simulink model "Simulator_swintheloop"  (R2016a)
settings: Solver=ode45  StartTime=0.0  StopTime=sim_time  RelTol=1e-3
values from neighbouring files (symbols this model uses):
  A_Servo = [0 1 0; 0 0 1 ; -B4/B1 -B3/B1 -B2/B1]    [Parameters.m]
  B_Servo = [0 ; 0 ; B0/B1]    [Parameters.m]
  C_Servo = eye(3)    [Parameters.m]
  delay_Kaltitude = 1    [Parameters.m]
  dLMN = [dLdp  0    0 ... (first row only)    [Parameters.m]
  g = 9.81    [Parameters.m]
  I_Pi = diag([8.450e-5 8.450e-5 4.580e-5])    [Parameters.m]
  In = diag([Ixx Iyy Izz])    [Parameters.m]
  InInv = In\eye(3)    [Parameters.m]
  KaD = 5.4    [Parameters.m]
  KaI = 3.6    [Parameters.m]
  KaN = 38    [Parameters.m]
  KaP = 8.0    (= 8)    [Parameters.m]
  Kba = sqrt(KaD/KaI)    [Parameters.m]
  Kbp = sqrt(Kdp/Kip)    [Parameters.m]
  Kbq = sqrt(Kdq/Kiq)    [Parameters.m]
  Kbr = sqrt(Kdr/Kir)    [Parameters.m]
  Kd_E = Kd_N    (= 0.01)    [Parameters.m]
  Kd_N = 0.01    [Parameters.m]
  Kd_u = Kd_v    (= 0.29)    [Parameters.m]
  Kd_v = 0.290    (= 0.29)    [Parameters.m]
  Kdp = 0.006    [Parameters.m]
  Kdq = Kdp    (= 0.006)    [Parameters.m]
  Kdr = 0.0153    [Parameters.m]
  Kinv = wpinv(K,W)    [Parameters.m]
  Kip = 0.72    [Parameters.m]
  Kiq = Kip    (= 0.72)    [Parameters.m]
  Kir = 0.125    [Parameters.m]
  Kp_E = Kp_N    (= 0.15)    [Parameters.m]
  Kp_N = 0.15    [Parameters.m]
  Kp_u = Kp_v    (= 6.3)    [Parameters.m]
  Kp_v = 6.3    [Parameters.m]
  KPD = KRD    (= 0.0584)    [Parameters.m]
  KPP = KRP    (= 1.61)    [Parameters.m]
  Kpp = 0.3    [Parameters.m]
  Kpq = Kpp    (= 0.3)    [Parameters.m]
  Kpr = 0.135    [Parameters.m]
  Kq = Cq*ro*A*R^3    (= 2.88925724261e-07)    [Parameters.m]
  KRD = 0.0584    [Parameters.m]
  KRP = 1.61    [Parameters.m]
  Kt = Ct*ro*A*R^2    (= 2.46191978476e-05)    [Parameters.m]
  m = 1.900    (= 1.9)    [Parameters.m]
  Mb = diag([m m m])    [Parameters.m]
  MbInv = Mb\eye(3)    [Parameters.m]
  N = 1/Tf    (= 100)    [Parameters.m]
  N_tras = 100    [Parameters.m]
  pitchMax = pi/6    (= 0.523598775598)    [Parameters.m]
  rollMax = pi/6    (= 0.523598775598)    [Parameters.m]
  satp = 1.5    [Parameters.m]
  satq = 1.5    [Parameters.m]
  satr = 1    [Parameters.m]
  tau = 0.055257    [Parameters.m]
  tc = 1/fc    (= 0.01)    [Parameters.m]
  x1 = [m q]    [Parameters.m]
  yawRateMax = pi/2    (= 1.57079632679)    [Parameters.m]
undefined symbols (not defined in the file or in its folder): Kp, KPI, KRI
libraries: simulink x10, aerolibutil x10
(part 2 of 2)

== system Simulator_swintheloop/TiltCopter/Actuators/Traslational Force_2 ==
  alpha_i : Inport
  omega_i : Inport  Port=2
  Product : Product  Multiplication=Matrix(*)
  R_BP2 : MATLAB Function  TreatAsAtomicUnit=on
  Thrust computation : Subsystem
  F_i : Outport
  wires:
  Thrust computation/1(Vector_Thrust_i) -> Product/2
  Product/1 -> F_i/1
  omega_i/1 -> Thrust computation/1(omega_i)
  R_BP2/1(Rotation_matrix) -> Product/1
  alpha_i/1 -> R_BP2/1(alpha_2)

== system Simulator_swintheloop/TiltCopter/Actuators/Traslational Force_3 ==
  alpha_i : Inport
  omega_i : Inport  Port=2
  Product : Product  Multiplication=Matrix(*)
  R_BP3 : MATLAB Function  TreatAsAtomicUnit=on
  Thrust computation : Subsystem
  F_i : Outport
  wires:
  Thrust computation/1(Vector_Thrust_i) -> Product/2
  Product/1 -> F_i/1
  omega_i/1 -> Thrust computation/1(omega_i)
  R_BP3/1(Rotation_matrix) -> Product/1
  alpha_i/1 -> R_BP3/1(alpha_3)

== system Simulator_swintheloop/TiltCopter/Actuators/Traslational Force_4 ==
  alpha_i : Inport
  omega_i : Inport  Port=2
  Product : Product  Multiplication=Matrix(*)
  R_BP4 : MATLAB Function  TreatAsAtomicUnit=on
  Thrust computation : Subsystem
  F_i : Outport
  wires:
  Thrust computation/1(Vector_Thrust_i) -> Product/2
  Product/1 -> F_i/1
  omega_i/1 -> Thrust computation/1(omega_i)
  R_BP4/1(Rotation_matrix) -> Product/1
  alpha_i/1 -> R_BP4/1(alpha_4)

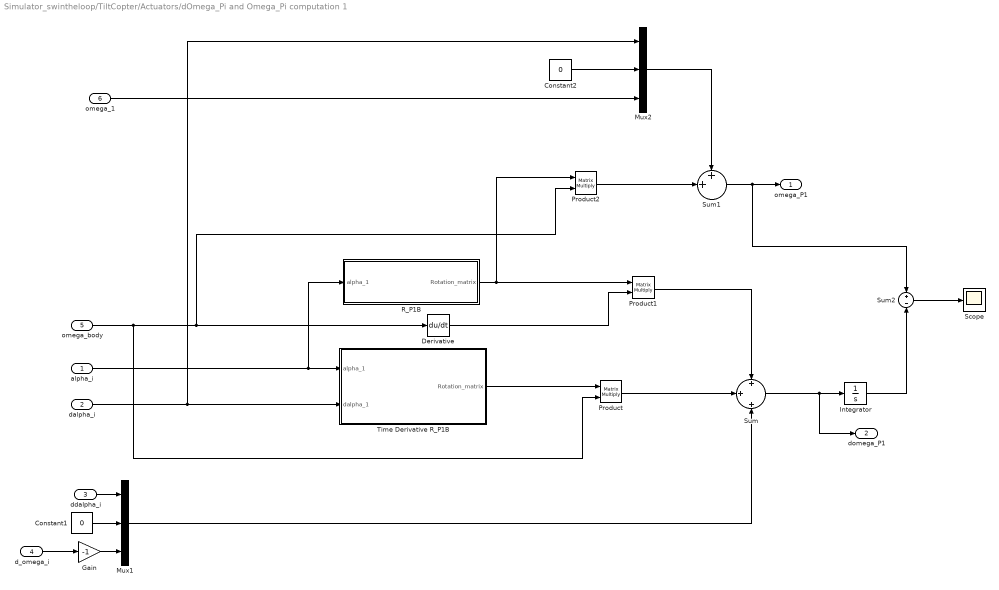
== system Simulator_swintheloop/TiltCopter/Actuators/dOmega_Pi and Omega_Pi computation 1 ==
  alpha_i : Inport
  dalpha_i : Inport  Port=2
  ddalpha_i : Inport  Port=3
  d_omega_i : Inport  Port=4
  omega_body : Inport  Port=5
  omega_1 : Inport  Port=6
  Constant1 : Constant  Value=0
  Constant2 : Constant  Value=0
  Derivative : Derivative
  Gain : Gain  Gain=-1
  Integrator : Integrator
  Mux1 : Mux  Inputs=3
  Mux2 : Mux  Inputs=3
  Product : Product  Multiplication=Matrix(*)
  Product1 : Product  Multiplication=Matrix(*)
  Product2 : Product  Multiplication=Matrix(*)
  R_P1B : MATLAB Function  TreatAsAtomicUnit=on
  Scope : Scope
  Sum : Sum  Inputs=+|+|+
  Sum1 : Sum  Inputs=++|
  Sum2 : Sum  Inputs=+-
  Time Derivative R_P1B : MATLAB Function  TreatAsAtomicUnit=on
  omega_P1 : Outport
  domega_P1 : Outport  Port=2
  wires:
  Derivative/1 -> Product1/2
  Product/1 -> Sum/2
  Time Derivative R_P1B/1(Rotation_matrix) -> Product/1
  Constant1/1 -> Mux1/2
  omega_body/1 -> Product/2, Product2/2, Derivative/1
  dalpha_i/1 -> Mux2/1, Time Derivative R_P1B/2(dalpha_1)
  alpha_i/1 -> R_P1B/1(alpha_1), Time Derivative R_P1B/1(alpha_1)
  R_P1B/1(Rotation_matrix) -> Product2/1, Product1/1
  Sum/1 -> domega_P1/1, Integrator/1
  Product1/1 -> Sum/1
  Mux1/1 -> Sum/3
  ddalpha_i/1 -> Mux1/1
  Product2/1 -> Sum1/2
  Constant2/1 -> Mux2/2
  Mux2/1 -> Sum1/1
  Sum1/1 -> Sum2/1, omega_P1/1
  omega_1/1 -> Mux2/3
  d_omega_i/1 -> Gain/1
  Integrator/1 -> Sum2/2
  Sum2/1 -> Scope/1
  Gain/1 -> Mux1/3

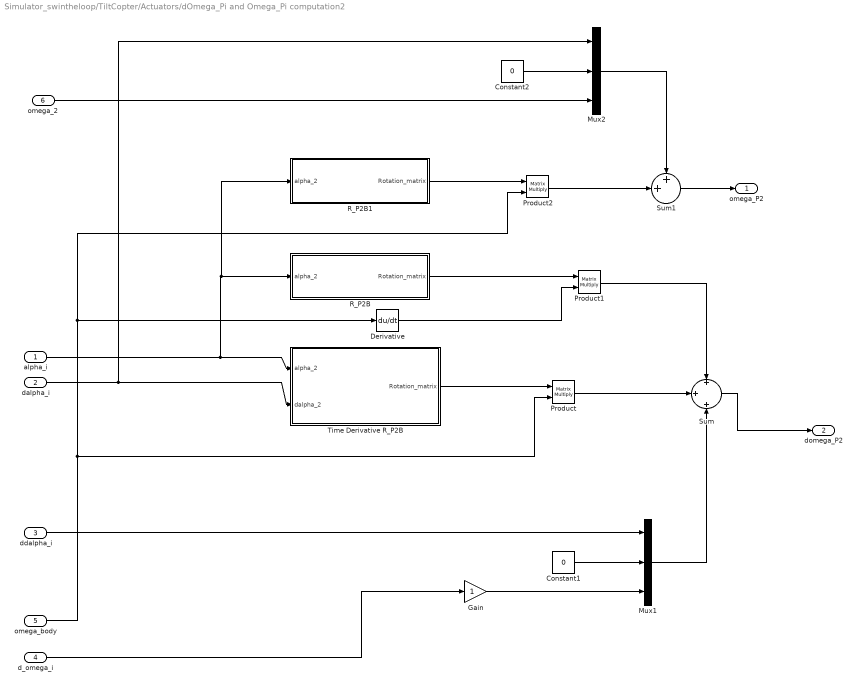
== system Simulator_swintheloop/TiltCopter/Actuators/dOmega_Pi and Omega_Pi computation2 ==
  alpha_i : Inport
  dalpha_i : Inport  Port=2
  ddalpha_i : Inport  Port=3
  d_omega_i : Inport  Port=4
  omega_body : Inport  Port=5
  omega_2 : Inport  Port=6
  Constant1 : Constant  Value=0
  Constant2 : Constant  Value=0
  Derivative : Derivative
  Gain : Gain
  Mux1 : Mux  Inputs=3
  Mux2 : Mux  Inputs=3
  Product : Product  Multiplication=Matrix(*)
  Product1 : Product  Multiplication=Matrix(*)
  Product2 : Product  Multiplication=Matrix(*)
  R_P2B : MATLAB Function  TreatAsAtomicUnit=on
  R_P2B1 : MATLAB Function  TreatAsAtomicUnit=on
  Sum : Sum  Inputs=+|+|+
  Sum1 : Sum  Inputs=++|
  Time Derivative R_P2B : MATLAB Function  TreatAsAtomicUnit=on
  omega_P2 : Outport
  domega_P2 : Outport  Port=2
  wires:
  Derivative/1 -> Product1/2
  Product/1 -> Sum/2
  Time Derivative R_P2B/1(Rotation_matrix) -> Product/1
  Constant1/1 -> Mux1/2
  omega_body/1 -> Product/2, Product2/2, Derivative/1
  dalpha_i/1 -> Mux2/1, Time Derivative R_P2B/2(dalpha_2)
  alpha_i/1 -> R_P2B1/1(alpha_2), R_P2B/1(alpha_2), Time Derivative R_P2B/1(alpha_2)
  Sum/1 -> domega_P2/1
  Product1/1 -> Sum/1
  Mux1/1 -> Sum/3
  ddalpha_i/1 -> Mux1/1
  R_P2B/1(Rotation_matrix) -> Product1/1
  R_P2B1/1(Rotation_matrix) -> Product2/1
  Product2/1 -> Sum1/2
  Constant2/1 -> Mux2/2
  Mux2/1 -> Sum1/1
  Sum1/1 -> omega_P2/1
  d_omega_i/1 -> Gain/1
  omega_2/1 -> Mux2/3
  Gain/1 -> Mux1/3

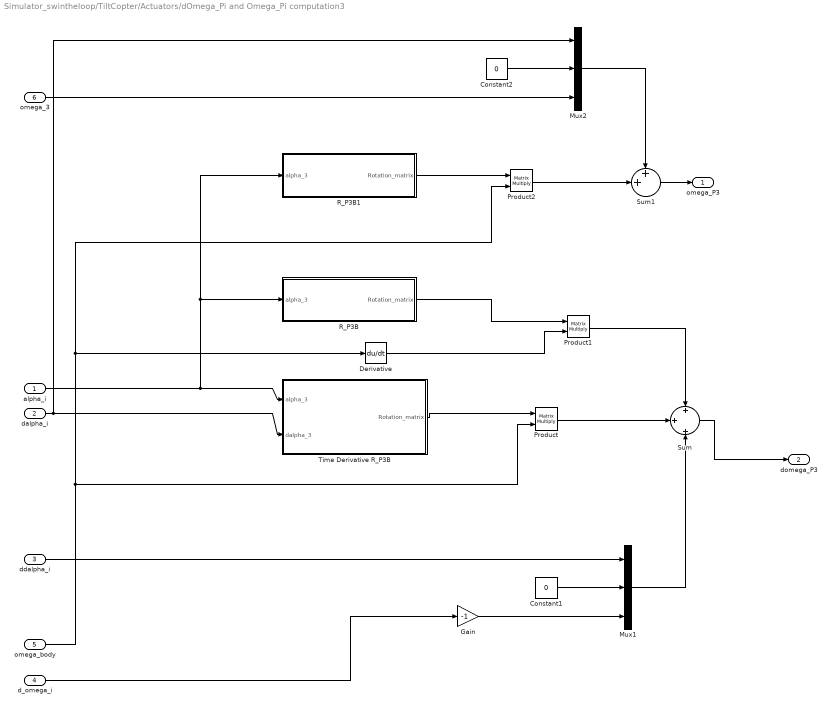
== system Simulator_swintheloop/TiltCopter/Actuators/dOmega_Pi and Omega_Pi computation3 ==
  alpha_i : Inport
  dalpha_i : Inport  Port=2
  ddalpha_i : Inport  Port=3
  d_omega_i : Inport  Port=4
  omega_body : Inport  Port=5
  omega_3 : Inport  Port=6
  Constant1 : Constant  Value=0
  Constant2 : Constant  Value=0
  Derivative : Derivative
  Gain : Gain  Gain=-1
  Mux1 : Mux  Inputs=3
  Mux2 : Mux  Inputs=3
  Product : Product  Multiplication=Matrix(*)
  Product1 : Product  Multiplication=Matrix(*)
  Product2 : Product  Multiplication=Matrix(*)
  R_P3B : MATLAB Function  TreatAsAtomicUnit=on
  R_P3B1 : MATLAB Function  TreatAsAtomicUnit=on
  Sum : Sum  Inputs=+|+|+
  Sum1 : Sum  Inputs=++|
  Time Derivative R_P3B : MATLAB Function  TreatAsAtomicUnit=on
  omega_P3 : Outport
  domega_P3 : Outport  Port=2
  wires:
  Derivative/1 -> Product1/2
  Product/1 -> Sum/2
  Time Derivative R_P3B/1(Rotation_matrix) -> Product/1
  Constant1/1 -> Mux1/2
  omega_body/1 -> Product/2, Product2/2, Derivative/1
  alpha_i/1 -> R_P3B1/1(alpha_3), R_P3B/1(alpha_3), Time Derivative R_P3B/1(alpha_3)
  Sum/1 -> domega_P3/1
  Product1/1 -> Sum/1
  Mux1/1 -> Sum/3
  ddalpha_i/1 -> Mux1/1
  R_P3B/1(Rotation_matrix) -> Product1/1
  R_P3B1/1(Rotation_matrix) -> Product2/1
  Product2/1 -> Sum1/2
  Constant2/1 -> Mux2/2
  Mux2/1 -> Sum1/1
  dalpha_i/1 -> Mux2/1, Time Derivative R_P3B/2(dalpha_3)
  Sum1/1 -> omega_P3/1
  d_omega_i/1 -> Gain/1
  omega_3/1 -> Mux2/3
  Gain/1 -> Mux1/3

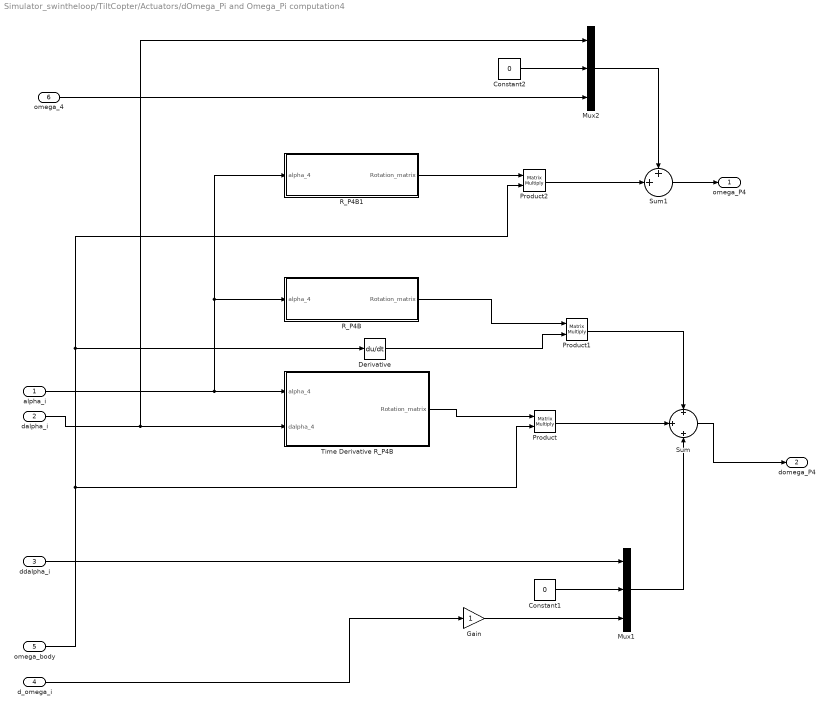
== system Simulator_swintheloop/TiltCopter/Actuators/dOmega_Pi and Omega_Pi computation4 ==
  alpha_i : Inport
  dalpha_i : Inport  Port=2
  ddalpha_i : Inport  Port=3
  d_omega_i : Inport  Port=4
  omega_body : Inport  Port=5
  omega_4 : Inport  Port=6
  Constant1 : Constant  Value=0
  Constant2 : Constant  Value=0
  Derivative : Derivative
  Gain : Gain
  Mux1 : Mux  Inputs=3
  Mux2 : Mux  Inputs=3
  Product : Product  Multiplication=Matrix(*)
  Product1 : Product  Multiplication=Matrix(*)
  Product2 : Product  Multiplication=Matrix(*)
  R_P4B : MATLAB Function  TreatAsAtomicUnit=on
  R_P4B1 : MATLAB Function  TreatAsAtomicUnit=on
  Sum : Sum  Inputs=+|+|+
  Sum1 : Sum  Inputs=++|
  Time Derivative R_P4B : MATLAB Function  TreatAsAtomicUnit=on
  omega_P4 : Outport
  domega_P4 : Outport  Port=2
  wires:
  Derivative/1 -> Product1/2
  Product/1 -> Sum/2
  Time Derivative R_P4B/1(Rotation_matrix) -> Product/1
  Constant1/1 -> Mux1/2
  omega_body/1 -> Product/2, Product2/2, Derivative/1
  dalpha_i/1 -> Mux2/1, Time Derivative R_P4B/2(dalpha_4)
  alpha_i/1 -> R_P4B1/1(alpha_4), R_P4B/1(alpha_4), Time Derivative R_P4B/1(alpha_4)
  Sum/1 -> domega_P4/1
  Product1/1 -> Sum/1
  Mux1/1 -> Sum/3
  ddalpha_i/1 -> Mux1/1
  R_P4B/1(Rotation_matrix) -> Product1/1
  Product2/1 -> Sum1/2
  Constant2/1 -> Mux2/2
  Mux2/1 -> Sum1/1
  R_P4B1/1(Rotation_matrix) -> Product2/1
  Sum1/1 -> omega_P4/1
  omega_4/1 -> Mux2/3
  d_omega_i/1 -> Gain/1
  Gain/1 -> Mux1/3

== system Simulator_swintheloop/TiltCopter/Actuators/tau_p1 computation ==
  omega_P1 : Inport
  domega_P1 : Inport  Port=2
  omega_i : Inport  Port=3
  3x3 Cross Product : aerolibutil/3x3 Cross Product
  Constant : Constant  Value=I_Pi
  Drag torque computation : Subsystem
  Gain : Gain  Gain=[1;1;1]
  Product : Product  Multiplication=Matrix(*)
  Product1 : Product  Multiplication=Matrix(*)
  Sum : Sum  Inputs=+|+|-
  tau_P1 : Outport
  wires:
  Constant/1 -> Product/1, Product1/1
  omega_P1/1 -> 3x3 Cross Product/1, Product1/2
  Product/1 -> Sum/2
  domega_P1/1 -> Product/2
  Product1/1 -> 3x3 Cross Product/2
  Sum/1 -> tau_P1/1
  3x3 Cross Product/1 -> Sum/1
  Drag torque computation/1(Vector_DragTorque_i) -> Gain/1
  omega_i/1 -> Drag torque computation/1(omega_P1_z)
  Gain/1 -> Sum/3

== system Simulator_swintheloop/TiltCopter/Actuators/tau_p2 computation ==
  omega_P2 : Inport
  domega_P2 : Inport  Port=2
  omega_i : Inport  Port=3
  3x3 Cross Product : aerolibutil/3x3 Cross Product
  Constant : Constant  Value=I_Pi
  Drag torque computation : Subsystem
  Gain : Gain  Gain=[1;1;1]
  Product : Product  Multiplication=Matrix(*)
  Product1 : Product  Multiplication=Matrix(*)
  Sum : Sum  Inputs=+|+|-
  tau_P2 : Outport
  wires:
  3x3 Cross Product/1 -> Sum/1
  Sum/1 -> tau_P2/1
  Product1/1 -> 3x3 Cross Product/2
  domega_P2/1 -> Product/2
  Product/1 -> Sum/2
  omega_P2/1 -> Product1/2, 3x3 Cross Product/1
  Constant/1 -> Product/1, Product1/1
  Drag torque computation/1(Vector_DragTorque_i) -> Gain/1
  omega_i/1 -> Drag torque computation/1(omega_P2)
  Gain/1 -> Sum/3

== system Simulator_swintheloop/TiltCopter/Actuators/tau_p3 computation1 ==
  omega_P3 : Inport
  domega_P3 : Inport  Port=2
  omega_i : Inport  Port=3
  3x3 Cross Product : aerolibutil/3x3 Cross Product
  Constant : Constant  Value=I_Pi
  Drag torque computation : Subsystem
  Gain : Gain  Gain=[1;1;1]
  Product : Product  Multiplication=Matrix(*)
  Product1 : Product  Multiplication=Matrix(*)
  Sum : Sum  Inputs=+|+|-
  tau_P3 : Outport
  wires:
  Constant/1 -> Product1/1, Product/1
  omega_P3/1 -> 3x3 Cross Product/1, Product1/2
  Product/1 -> Sum/2
  domega_P3/1 -> Product/2
  Product1/1 -> 3x3 Cross Product/2
  Sum/1 -> tau_P3/1
  3x3 Cross Product/1 -> Sum/1
  Drag torque computation/1(Vector_DragTorque_i) -> Gain/1
  omega_i/1 -> Drag torque computation/1(omega_P3)
  Gain/1 -> Sum/3

== system Simulator_swintheloop/TiltCopter/Actuators/tau_p4 computation2 ==
  omega_P4 : Inport
  domega_P4 : Inport  Port=2
  omega_i : Inport  Port=3
  3x3 Cross Product : aerolibutil/3x3 Cross Product
  Constant : Constant  Value=I_Pi
  Drag torque computation : Subsystem
  Gain : Gain  Gain=[1;1;1]
  Product : Product  Multiplication=Matrix(*)
  Product1 : Product  Multiplication=Matrix(*)
  Sum : Sum  Inputs=+|+|-
  tau_P4 : Outport
  wires:
  3x3 Cross Product/1 -> Sum/1
  Sum/1 -> tau_P4/1
  Product1/1 -> 3x3 Cross Product/2
  domega_P4/1 -> Product/2
  Product/1 -> Sum/2
  omega_P4/1 -> Product1/2, 3x3 Cross Product/1
  Constant/1 -> Product/1, Product1/1
  Drag torque computation/1(Vector_DragTorque_i) -> Gain/1
  omega_i/1 -> Drag torque computation/1(omega_P4)
  Gain/1 -> Sum/3

== system Simulator_swintheloop/TiltCopter/Actuators/ESC+Brushless1/Subsystem ==
  Throttle [%] : Inport
  Bias : Bias  Bias=x1(2)
  Gain : Gain  Gain=x1(1)
  Gain1 : Gain  Gain=-1/tau
  Gain2 : Gain  Gain=1/tau
  Gain3 : Gain  Gain=x1(1)
  Gain4 : Gain  Gain=x1(1)
  Sum : Sum  Inputs=|++
  Transfer Fcn : TransferFcn  Denominator=[(tau) 1]
  Transfer Fcn1 : TransferFcn  Denominator=[(tau) 1]
  omega_i : Outport
  domega_i : Outport  Port=2
  wires:
  Throttle [%]/1 -> Gain4/1, Transfer Fcn1/1, Transfer Fcn/1
  Transfer Fcn1/1 -> Gain1/1
  Gain1/1 -> Gain3/1
  Sum/1 -> domega_i/1
  Gain2/1 -> Sum/2
  Gain3/1 -> Sum/1
  Bias/1 -> omega_i/1
  Gain/1 -> Bias/1
  Transfer Fcn/1 -> Gain/1
  Gain4/1 -> Gain2/1

== system Simulator_swintheloop/TiltCopter/Actuators/ESC+Brushless2/Subsystem ==
  Throttle [%] : Inport
  Bias : Bias  Bias=x1(2)
  Gain : Gain  Gain=x1(1)
  Gain1 : Gain  Gain=-1/tau
  Gain2 : Gain  Gain=1/tau
  Gain3 : Gain  Gain=x1(1)
  Gain4 : Gain  Gain=x1(1)
  Sum : Sum  Inputs=|++
  Transfer Fcn : TransferFcn  Denominator=[(tau) 1]
  Transfer Fcn1 : TransferFcn  Denominator=[(tau) 1]
  omega_i : Outport
  domega_i : Outport  Port=2
  wires:
  Throttle [%]/1 -> Gain4/1, Transfer Fcn1/1, Transfer Fcn/1
  Transfer Fcn1/1 -> Gain1/1
  Gain1/1 -> Gain3/1
  Sum/1 -> domega_i/1
  Gain2/1 -> Sum/2
  Gain3/1 -> Sum/1
  Bias/1 -> omega_i/1
  Gain/1 -> Bias/1
  Transfer Fcn/1 -> Gain/1
  Gain4/1 -> Gain2/1

== system Simulator_swintheloop/TiltCopter/Actuators/ESC+Brushless3/Subsystem ==
  Throttle [%] : Inport
  Bias : Bias  Bias=x1(2)
  Gain : Gain  Gain=x1(1)
  Gain1 : Gain  Gain=-1/tau
  Gain2 : Gain  Gain=1/tau
  Gain3 : Gain  Gain=x1(1)
  Gain4 : Gain  Gain=x1(1)
  Sum : Sum  Inputs=|++
  Transfer Fcn : TransferFcn  Denominator=[(tau) 1]
  Transfer Fcn1 : TransferFcn  Denominator=[(tau) 1]
  omega_i : Outport
  domega_i : Outport  Port=2
  wires:
  Throttle [%]/1 -> Gain4/1, Transfer Fcn1/1, Transfer Fcn/1
  Transfer Fcn1/1 -> Gain1/1
  Gain1/1 -> Gain3/1
  Sum/1 -> domega_i/1
  Gain2/1 -> Sum/2
  Gain3/1 -> Sum/1
  Bias/1 -> omega_i/1
  Gain/1 -> Bias/1
  Transfer Fcn/1 -> Gain/1
  Gain4/1 -> Gain2/1

== system Simulator_swintheloop/TiltCopter/Actuators/ESC+Brushless4/Subsystem ==
  Throttle [%] : Inport
  Bias : Bias  Bias=x1(2)
  Gain : Gain  Gain=x1(1)
  Gain1 : Gain  Gain=-1/tau
  Gain2 : Gain  Gain=1/tau
  Gain3 : Gain  Gain=x1(1)
  Gain4 : Gain  Gain=x1(1)
  Sum : Sum  Inputs=|++
  Transfer Fcn : TransferFcn  Denominator=[(tau) 1]
  Transfer Fcn1 : TransferFcn  Denominator=[(tau) 1]
  omega_i : Outport
  domega_i : Outport  Port=2
  wires:
  Throttle [%]/1 -> Gain4/1, Transfer Fcn1/1, Transfer Fcn/1
  Transfer Fcn1/1 -> Gain1/1
  Gain1/1 -> Gain3/1
  Sum/1 -> domega_i/1
  Gain2/1 -> Sum/2
  Gain3/1 -> Sum/1
  Bias/1 -> omega_i/1
  Gain/1 -> Bias/1
  Transfer Fcn/1 -> Gain/1
  Gain4/1 -> Gain2/1

== system Simulator_swintheloop/TiltCopter/Actuators/External Momentum_1/Thrust computation ==
  omega_i : Inport
  Constant : Constant  Value=-Kt
  Constant1 : Constant  Value=0
  Constant2 : Constant  Value=0
  Mux : Mux  Inputs=3
  Product : Product
  Product1 : Product
  Vector_Thrust_i : Outport
  wires:
  Constant2/1 -> Mux/2
  omega_i/1 -> Product/2, Product/1
  Product/1 -> Product1/1
  Constant1/1 -> Mux/1
  Mux/1 -> Vector_Thrust_i/1
  Product1/1 -> Mux/3
  Constant/1 -> Product1/2

== system Simulator_swintheloop/TiltCopter/Actuators/External Momentum_2/Thrust computation ==
  omega_i : Inport
  Constant : Constant  Value=-Kt
  Constant1 : Constant  Value=0
  Constant2 : Constant  Value=0
  Mux : Mux  Inputs=3
  Product : Product
  Product1 : Product
  Vector_Thrust_i : Outport
  wires:
  Constant2/1 -> Mux/2
  omega_i/1 -> Product/2, Product/1
  Product/1 -> Product1/1
  Constant1/1 -> Mux/1
  Mux/1 -> Vector_Thrust_i/1
  Product1/1 -> Mux/3
  Constant/1 -> Product1/2

== system Simulator_swintheloop/TiltCopter/Actuators/External Momentum_3/Thrust computation ==
  omega_i : Inport
  Constant : Constant  Value=-Kt
  Constant1 : Constant  Value=0
  Constant2 : Constant  Value=0
  Mux : Mux  Inputs=3
  Product : Product
  Product1 : Product
  Vector_Thrust_i : Outport
  wires:
  Constant2/1 -> Mux/2
  omega_i/1 -> Product/2, Product/1
  Product/1 -> Product1/1
  Constant1/1 -> Mux/1
  Mux/1 -> Vector_Thrust_i/1
  Product1/1 -> Mux/3
  Constant/1 -> Product1/2

== system Simulator_swintheloop/TiltCopter/Actuators/External Momentum_4/Thrust computation ==
  omega_i : Inport
  Constant : Constant  Value=-Kt
  Constant1 : Constant  Value=0
  Constant2 : Constant  Value=0
  Mux : Mux  Inputs=3
  Product : Product
  Product1 : Product
  Vector_Thrust_i : Outport
  wires:
  Constant2/1 -> Mux/2
  omega_i/1 -> Product/2, Product/1
  Product/1 -> Product1/1
  Constant1/1 -> Mux/1
  Mux/1 -> Vector_Thrust_i/1
  Product1/1 -> Mux/3
  Constant/1 -> Product1/2

== system Simulator_swintheloop/TiltCopter/Actuators/Traslational Force_1/Thrust computation ==
  omega_i : Inport
  Constant : Constant  Value=-Kt
  Constant1 : Constant  Value=0
  Constant2 : Constant  Value=0
  Mux : Mux  Inputs=3
  Product : Product
  Product1 : Product
  Vector_Thrust_i : Outport
  wires:
  Constant2/1 -> Mux/2
  omega_i/1 -> Product/2, Product/1
  Product/1 -> Product1/1
  Constant1/1 -> Mux/1
  Mux/1 -> Vector_Thrust_i/1
  Product1/1 -> Mux/3
  Constant/1 -> Product1/2

== system Simulator_swintheloop/TiltCopter/Actuators/Traslational Force_2/Thrust computation ==
  omega_i : Inport
  Constant : Constant  Value=-Kt
  Constant1 : Constant  Value=0
  Constant2 : Constant  Value=0
  Mux : Mux  Inputs=3
  Product : Product
  Product1 : Product
  Vector_Thrust_i : Outport
  wires:
  Constant2/1 -> Mux/2
  omega_i/1 -> Product/2, Product/1
  Product/1 -> Product1/1
  Constant1/1 -> Mux/1
  Mux/1 -> Vector_Thrust_i/1
  Product1/1 -> Mux/3
  Constant/1 -> Product1/2

== system Simulator_swintheloop/TiltCopter/Actuators/Traslational Force_3/Thrust computation ==
  omega_i : Inport
  Constant : Constant  Value=-Kt
  Constant1 : Constant  Value=0
  Constant2 : Constant  Value=0
  Mux : Mux  Inputs=3
  Product : Product
  Product1 : Product
  Vector_Thrust_i : Outport
  wires:
  Constant2/1 -> Mux/2
  omega_i/1 -> Product/2, Product/1
  Product/1 -> Product1/1
  Constant1/1 -> Mux/1
  Mux/1 -> Vector_Thrust_i/1
  Product1/1 -> Mux/3
  Constant/1 -> Product1/2

== system Simulator_swintheloop/TiltCopter/Actuators/Traslational Force_4/Thrust computation ==
  omega_i : Inport
  Constant : Constant  Value=-Kt
  Constant1 : Constant  Value=0
  Constant2 : Constant  Value=0
  Mux : Mux  Inputs=3
  Product : Product
  Product1 : Product
  Vector_Thrust_i : Outport
  wires:
  Constant2/1 -> Mux/2
  omega_i/1 -> Product/2, Product/1
  Product/1 -> Product1/1
  Constant1/1 -> Mux/1
  Mux/1 -> Vector_Thrust_i/1
  Product1/1 -> Mux/3
  Constant/1 -> Product1/2

== system Simulator_swintheloop/TiltCopter/Actuators/tau_p1 computation/Drag torque computation ==
  omega_P1_z : Inport
  Constant : Constant  Value=-Kq
  Constant1 : Constant  Value=0
  Constant2 : Constant  Value=0
  Mux : Mux  Inputs=3
  Product : Product
  Product1 : Product
  Vector_DragTorque_i : Outport
  wires:
  Constant2/1 -> Mux/2
  Product/1 -> Product1/1
  Constant1/1 -> Mux/1
  Mux/1 -> Vector_DragTorque_i/1
  Product1/1 -> Mux/3
  Constant/1 -> Product1/2
  omega_P1_z/1 -> Product/2, Product/1

== system Simulator_swintheloop/TiltCopter/Actuators/tau_p2 computation/Drag torque computation ==
  omega_P2 : Inport
  Constant : Constant  Value=Kq
  Constant1 : Constant  Value=0
  Constant2 : Constant  Value=0
  Mux : Mux  Inputs=3
  Product : Product
  Product1 : Product
  Vector_DragTorque_i : Outport
  wires:
  Constant2/1 -> Mux/2
  Product/1 -> Product1/1
  Constant1/1 -> Mux/1
  Mux/1 -> Vector_DragTorque_i/1
  Product1/1 -> Mux/3
  Constant/1 -> Product1/2
  omega_P2/1 -> Product/2, Product/1

== system Simulator_swintheloop/TiltCopter/Actuators/tau_p3 computation1/Drag torque computation ==
  omega_P3 : Inport
  Constant : Constant  Value=-Kq
  Constant1 : Constant  Value=0
  Constant2 : Constant  Value=0
  Mux : Mux  Inputs=3
  Product : Product
  Product1 : Product
  Vector_DragTorque_i : Outport
  wires:
  Constant2/1 -> Mux/2
  Product/1 -> Product1/1
  Constant1/1 -> Mux/1
  Mux/1 -> Vector_DragTorque_i/1
  Product1/1 -> Mux/3
  Constant/1 -> Product1/2
  omega_P3/1 -> Product/2, Product/1

== system Simulator_swintheloop/TiltCopter/Actuators/tau_p4 computation2/Drag torque computation ==
  omega_P4 : Inport
  Constant : Constant  Value=Kq
  Constant1 : Constant  Value=0
  Constant2 : Constant  Value=0
  Mux : Mux  Inputs=3
  Product : Product
  Product1 : Product
  Vector_DragTorque_i : Outport
  wires:
  Constant2/1 -> Mux/2
  Product/1 -> Product1/1
  Constant1/1 -> Mux/1
  Mux/1 -> Vector_DragTorque_i/1
  Product1/1 -> Mux/3
  Constant/1 -> Product1/2
  omega_P4/1 -> Product/2, Product/1

== matlab function Simulator_swintheloop/TiltCopter/To body from Earth ==
  data: Alpha_e input; Earth input; body output
 function body = Tbe(Alpha_e, Earth)
%#codegen
phi = Alpha_e(1);
theta = Alpha_e(2);
psi = Alpha_e(3);

Sphi = sin(phi);
Cphi = cos(phi);
Stheta = sin(theta);
Ctheta = cos(theta);
Spsi = sin(psi);
Cpsi = cos(psi);

TBE = [        Ctheta*Cpsi               Ctheta*Spsi          -Stheta    ;
       Sphi*Stheta*Cpsi-Cphi*Spsi Sphi*Stheta*Spsi+Cphi*Cpsi Sphi*Ctheta ;
       Cphi*Stheta*Cpsi+Sphi*Spsi Cphi*Stheta*Spsi-Sphi*Cpsi Cphi*Ctheta];

body = TBE* Earth;

== matlab function Simulator_swintheloop/TiltCopter/To Earth from body ==
  data: Alpha_e input; Earth output; body input
 function Earth = Tbet(Alpha_e, body)
%#codegen
phi = Alpha_e(1);
theta = Alpha_e(2);
psi = Alpha_e(3);

Sphi = sin(phi);
Cphi = cos(phi);
Stheta = sin(theta);
Ctheta = cos(theta);
Spsi = sin(psi);
Cpsi = cos(psi);

TBE = [        Ctheta*Cpsi               Ctheta*Spsi          -Stheta    ;
       Sphi*Stheta*Cpsi-Cphi*Spsi Sphi*Stheta*Spsi+Cphi*Cpsi Sphi*Ctheta ;
       Cphi*Stheta*Cpsi+Sphi*Spsi Cphi*Stheta*Spsi-Sphi*Cpsi Cphi*Ctheta];
TEB = TBE';

Earth = TEB* body;

== matlab function Simulator_swintheloop/TiltCopter/To Earth from body_rates ==
  data: Alpha_e input; Rates_B input; Rates_E output
 function Rates_E = Einv(Alpha_e, Rates_B)
%#codegen
phi = Alpha_e(1);
theta = Alpha_e(2);

Sphi = sin(phi);
Cphi = cos(phi);
Ctheta = cos(theta);
Ttheta = tan(theta);

Einv = [1   Sphi*Ttheta    Cphi*Ttheta ;
        0       Cphi          -Sphi    ;
        0   Sphi/Ctheta    Cphi/Ctheta];

Rates_E = Einv* Rates_B;

== matlab function Simulator_swintheloop/TiltCopter/Actuators/Traslational Force_1/R_BP1 ==
  data: Rotation_matrix output; alpha_1 input
function Rotation_matrix = fcn(alpha_1)
%#codegen

% Rotation matrix from group propeller 1 to body
R_BP1 = [ 1,0,0; 0, cos(alpha_1), -sin(alpha_1);0, sin(alpha_1),cos(alpha_1)];
      



Rotation_matrix = R_BP1;

== matlab function Simulator_swintheloop/Controllers/Attitude Controller/To body from Earth_rates ==
  data: Alpha_e input; Rates_B output; Rates_E input
 function Rates_B = E(Alpha_e, Rates_E)
%#codegen
phi = Alpha_e(1);       % Roll
theta = Alpha_e(2);     % Pitch
psi = Alpha_e(3);       % Yaw

E = [cos(psi)*cos(theta),cos(theta)*sin(psi),-sin(theta);
 cos(psi)*sin(phi)*sin(theta) - cos(phi)*sin(psi), cos(phi)*cos(psi) + sin(phi)*sin(psi)*sin(theta), cos(theta)*sin(phi);
 sin(phi)*sin(psi) + cos(phi)*cos(psi)*sin(theta), cos(phi)*sin(psi)*sin(theta) - cos(psi)*sin(phi), cos(phi)*cos(theta)];

Rates_B = E* Rates_E;

== matlab function Simulator_swintheloop/Controllers/Position Controller Tilt/NED to body ==
  data: pos_x output; pos_y output; pos_z output; phi input; theta input; psi input; pos_n input; pos_e input; pos_d input
function [pos_x,pos_y,pos_z] = ned2body(phi,theta,psi,pos_n,pos_e,pos_d)
%#codegen
Pos_NED = [pos_n ;
    pos_e ;
    pos_d];

%% Rotate Acc_body to Earth frame
Sphi = sin(phi);
Cphi = cos(phi);
Stheta = sin(theta);
Ctheta = cos(theta);
Spsi = sin(psi);
Cpsi = cos(psi);

Tbe = [           Cpsi*Ctheta,                  Ctheta*Spsi,     -Stheta;
 Cpsi*Sphi*Stheta - Cphi*Spsi, Cphi*Cpsi + Sphi*Spsi*Stheta, Ctheta*Sphi;
 Sphi*Spsi + Cphi*Cpsi*Stheta, Cphi*Spsi*Stheta - Cpsi*Sphi, Cphi*Ctheta];

Tbet = [ Cpsi*Ctheta, Cpsi*Sphi*Stheta - Cphi*Spsi, Sphi*Spsi + Cphi*Cpsi*Stheta ;
         Ctheta*Spsi, Cphi*Cpsi + Sphi*Spsi*Stheta, Cphi*Spsi*Stheta - Cpsi*Sphi ;
             -Stheta,                  Ctheta*Sphi,                  Cphi*Ctheta];

% Acc_Earth = zeros(3,1);

Pos_body = Tbe * Pos_NED ;

pos_x = Pos_body(1);
pos_y = Pos_body(2);
pos_z = Pos_body(3);

== matlab function Simulator_swintheloop/TiltCopter/Actuators/dOmega_Pi and Omega_Pi computation 1/Time Derivative R_P1B ==
  data: alpha_1 input; dalpha_1 input; Rotation_matrix output
function Rotation_matrix = fcn(alpha_1,dalpha_1)
%#codegen
dR_P1B = [ 0 0 0 ; 
          0 -sin(alpha_1) cos(alpha_1);
          0 -cos(alpha_1) -sin(alpha_1)];
      
Rotation_matrix = dR_P1B*dalpha_1;

== matlab function Simulator_swintheloop/TiltCopter/Actuators/dOmega_Pi and Omega_Pi computation2/Time Derivative R_P2B ==
  data: alpha_2 input; dalpha_2 input; Rotation_matrix output
function Rotation_matrix = fcn(alpha_2,dalpha_2)
%#codegen
% omega_x = -dalpha_i;
% omega_y = 0;
% omega_z = 0;
% Define the skew simmetric matrix
% S = [0 -omega_z omega_y;omega_z 0 -omega_x; -omega_y omega_x 0];


%Time derivative of Rotation matrix from Body to propeller group 1
% This rotation matrix is obtained with the Skew symmetric matrix
% In fact R_dot = S(alpha) * R_BPi

dR_P2B = [ 0 0 0 ; sin(alpha_2) 0 cos(alpha_2);...
           cos(alpha_2) 0 -sin(alpha_2)];
      
Rotation_matrix = dR_P2B*dalpha_2;

== matlab function Simulator_swintheloop/TiltCopter/Actuators/dOmega_Pi and Omega_Pi computation3/Time Derivative R_P3B ==
  data: alpha_3 input; dalpha_3 input; Rotation_matrix output
function Rotation_matrix = fcn(alpha_3,dalpha_3)
%#codegen
dR_P3B =[ 0 0 0 ; 0 sin(alpha_3) cos(alpha_3); 0 cos(alpha_3) -sin(alpha_3)]; 
      
Rotation_matrix = dR_P3B*dalpha_3;

== matlab function Simulator_swintheloop/TiltCopter/Actuators/Traslational Force_2/R_BP2 ==
  data: Rotation_matrix output; alpha_2 input
function Rotation_matrix = fcn(alpha_2)
%#codegen

% Rotation matrix from Propeller group 2 to body
R_BP2 =[ 0, -cos(alpha_2), sin(alpha_2); 1,0,0; 0,sin(alpha_2),cos(alpha_2)];

Rotation_matrix =R_BP2;

== matlab function Simulator_swintheloop/TiltCopter/Actuators/Traslational Force_3/R_BP3 ==
  data: Rotation_matrix output; alpha_3 input
function Rotation_matrix = fcn(alpha_3)
%#codegen

R_BP3 = [ -1, 0, 0;0, -cos(alpha_3), sin(alpha_3);0,  sin(alpha_3), cos(alpha_3)];

Rotation_matrix = R_BP3;

== matlab function Simulator_swintheloop/TiltCopter/Actuators/Traslational Force_4/R_BP4 ==
  data: Rotation_matrix output; alpha_4 input
function Rotation_matrix = fcn(alpha_4)
%#codegen

R_BP4 = [0, cos(alpha_4), -sin(alpha_4); -1, 0, 0; 0, sin(alpha_4), cos(alpha_4)];

Rotation_matrix = R_BP4;

== matlab function Simulator_swintheloop/TiltCopter/Actuators/dOmega_Pi and Omega_Pi computation4/Time Derivative R_P4B ==
  data: alpha_4 input; dalpha_4 input; Rotation_matrix output
function Rotation_matrix = fcn(alpha_4,dalpha_4)
%#codegen
dR_P4B = [ 0 0 0 ; -sin(alpha_4) 0 cos(alpha_4); -cos(alpha_4) 0 -sin(alpha_4)];
Rotation_matrix = dR_P4B*dalpha_4;

== matlab function Simulator_swintheloop/TiltCopter/Actuators/External Momentum_1/O_BPi ==
  data: Origin_Rotation output; motor_number input; b parameter
function Origin_Rotation = fcn(motor_number,b)
%#codegen

% Rotation matrix from Body to propeller group
psi = (motor_number-1)*pi/2;


R_z = [cos(psi), -sin(psi), 0;
      sin(psi),  cos(psi), 0;
      0,         0, 1];
      



Origin_Rotation = R_z*[b;0;0];

== matlab function Simulator_swintheloop/TiltCopter/Actuators/External Momentum_1/R_BP1 ==
  data: Rotation_matrix output; alpha_1 input
function Rotation_matrix = fcn(alpha_1)
%#codegen

% Rotation matrix from group propeller 1 to body
R_BP1 = [ 1,0,0; 0, cos(alpha_1), -sin(alpha_1);0, sin(alpha_1),cos(alpha_1)];
      



Rotation_matrix = R_BP1;

== matlab function Simulator_swintheloop/TiltCopter/Actuators/External Momentum_2/O_BPi ==
  data: Origin_Rotation output; motor_number input; b parameter
function Origin_Rotation = fcn(motor_number,b)
%#codegen

% Rotation matrix from Body to propeller group
psi = (motor_number-1)*pi/2;


R_z =[ cos(psi), -sin(psi), 0;
      sin(psi),  cos(psi), 0;
      0,         0, 1];
      



Origin_Rotation = R_z*[b;0;0];

== matlab function Simulator_swintheloop/TiltCopter/Actuators/External Momentum_2/R_BP2 ==
  data: Rotation_matrix output; alpha_2 input
function Rotation_matrix = fcn(alpha_2)
%#codegen

% Rotation matrix from Propeller group 2 to body
R_BP2 =[ 0, -cos(alpha_2), sin(alpha_2); 1,0,0; 0,sin(alpha_2),cos(alpha_2)];

Rotation_matrix =R_BP2;

== matlab function Simulator_swintheloop/TiltCopter/Actuators/External Momentum_3/O_BPi ==
  data: Origin_Rotation output; motor_number input; b parameter
function Origin_Rotation = fcn(motor_number,b)
%#codegen

% Rotation matrix from Body to propeller group
psi = (motor_number-1)*pi/2;


R_z = [cos(psi), -sin(psi), 0;
      sin(psi),  cos(psi), 0;
      0,         0, 1];
      



Origin_Rotation = R_z*[b;0;0];

== matlab function Simulator_swintheloop/TiltCopter/Actuators/External Momentum_3/R_BP3 ==
  data: Rotation_matrix output; alpha_3 input
function Rotation_matrix = fcn(alpha_3)
%#codegen

R_BP3 = [ -1, 0, 0;0, -cos(alpha_3), sin(alpha_3);0,  sin(alpha_3), cos(alpha_3)];

Rotation_matrix = R_BP3;

== matlab function Simulator_swintheloop/TiltCopter/Actuators/External Momentum_4/O_BPi ==
  data: Origin_Rotation output; motor_number input; b parameter
function Origin_Rotation = fcn(motor_number,b)
%#codegen

% Rotation matrix from Body to propeller group
psi = (motor_number-1)*pi/2;


R_z = [cos(psi), -sin(psi), 0;
      sin(psi),  cos(psi), 0;
      0,         0, 1];
      



Origin_Rotation = R_z*[b;0;0];

== matlab function Simulator_swintheloop/TiltCopter/Actuators/External Momentum_4/R_BP4 ==
  data: Rotation_matrix output; alpha_4 input
function Rotation_matrix = fcn(alpha_4)
%#codegen

R_BP4 = [0, cos(alpha_4), -sin(alpha_4); -1, 0, 0; 0, sin(alpha_4), cos(alpha_4)];

Rotation_matrix = R_BP4;

== matlab function Simulator_swintheloop/TiltCopter/Actuators/dOmega_Pi and Omega_Pi computation2/R_P2B ==
  data: alpha_2 input; Rotation_matrix output
function Rotation_matrix = fcn(alpha_2)
%#codegen
R_P2B = [0 1 0; -cos(alpha_2) 0 sin(alpha_2);sin(alpha_2) 0 cos(alpha_2)];
      
Rotation_matrix = R_P2B;

== matlab function Simulator_swintheloop/TiltCopter/Actuators/dOmega_Pi and Omega_Pi computation3/R_P3B ==
  data: alpha_3 input; Rotation_matrix output
function Rotation_matrix = fcn(alpha_3)
%#codegen
R_P3B = [ -1 0 0 ; 0 -cos(alpha_3) sin(alpha_3); 0 sin(alpha_3) cos(alpha_3)];
      
Rotation_matrix = R_P3B;

== matlab function Simulator_swintheloop/TiltCopter/Actuators/dOmega_Pi and Omega_Pi computation 1/R_P1B ==
  data: alpha_1 input; Rotation_matrix output
function Rotation_matrix = fcn(alpha_1)
%#codegen
R_P1B = [ 1 0 0 ; 0 cos(alpha_1) sin(alpha_1); 0 -sin(alpha_1) cos(alpha_1)];
      
Rotation_matrix = R_P1B;

== matlab function Simulator_swintheloop/TiltCopter/Actuators/dOmega_Pi and Omega_Pi computation4/R_P4B ==
  data: alpha_4 input; Rotation_matrix output
function Rotation_matrix = fcn(alpha_4)
%#codegen
R_P4B = [0 -1 0; cos(alpha_4) 0 sin(alpha_4); -sin(alpha_4) 0 cos(alpha_4)];
      
Rotation_matrix = R_P4B;

== matlab function Simulator_swintheloop/TiltCopter/Actuators/dOmega_Pi and Omega_Pi computation2/R_P2B1 ==
  data: alpha_2 input; Rotation_matrix output
function Rotation_matrix = fcn(alpha_2)
%#codegen
R_P2B = [0 1 0; -cos(alpha_2) 0 sin(alpha_2);sin(alpha_2) 0 cos(alpha_2)];
      
Rotation_matrix = R_P2B;

== matlab function Simulator_swintheloop/TiltCopter/Actuators/dOmega_Pi and Omega_Pi computation3/R_P3B1 ==
  data: alpha_3 input; Rotation_matrix output
function Rotation_matrix = fcn(alpha_3)
%#codegen
R_P3B = [ -1 0 0 ; 0 -cos(alpha_3) sin(alpha_3); 0 sin(alpha_3) cos(alpha_3)];
      
Rotation_matrix = R_P3B;

== matlab function Simulator_swintheloop/TiltCopter/Actuators/dOmega_Pi and Omega_Pi computation4/R_P4B1 ==
  data: alpha_4 input; Rotation_matrix output
function Rotation_matrix = fcn(alpha_4)
%#codegen
R_P4B = [0 -1 0; cos(alpha_4) 0 sin(alpha_4); -sin(alpha_4) 0 cos(alpha_4)];
      
Rotation_matrix = R_P4B;
